simulink model "ET223104_complex_lab"  (R2023a)
settings: Solver=VariableStepAuto  StartTime=0.0  StopTime=10.0  RelTol=1e-3
libraries: spsThreePhaseSeriesRLCBranchLib x10, spsLoadFlowBusLib x9, spsThreePhaseVIMeasurementLib x9, spsThreePhaseParallelRLCLoadLib x6, spsThreePhaseSourceLib x3, sps_lib x1
settings Model: Creator=shahrearhossain  LastModifiedBy=shahrearhossain

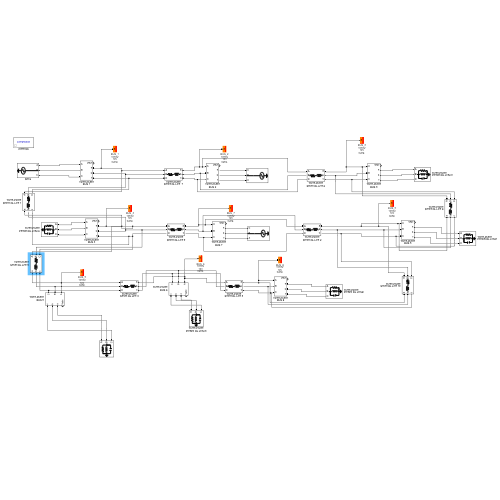
[thumbnail: Simulink's stored preview of the top-level diagram]
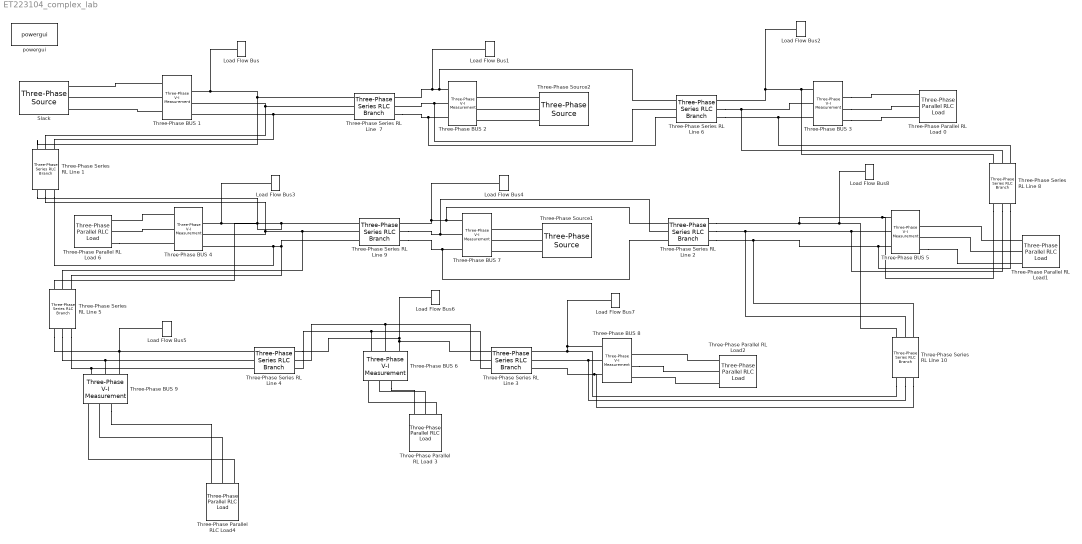
== system ET223104_complex_lab ==
  Load Flow Bus : spsLoadFlowBusLib/Load Flow Bus  LConnTagsString=a  Phases=single  Connectors=on one side  ID=BUS_1  Vbase=10e3  Vref=1.0  Vangle=0  VLF=1  VLFb=1  VLFc=1  angleLF=0  angleLFb=0  angleLFc=0
  Load Flow Bus1 : spsLoadFlowBusLib/Load Flow Bus  LConnTagsString=a  Phases=single  Connectors=on one side  ID=BUS_2  Vbase=10e3  Vref=1.05  Vangle=0  VLF=1  VLFb=1  VLFc=1  angleLF=0  angleLFb=0  angleLFc=0
  Load Flow Bus2 : spsLoadFlowBusLib/Load Flow Bus  LConnTagsString=a  Phases=single  Connectors=on one side  ID=BUS_3  Vbase=10e3  Vref=1.05  Vangle=0  VLF=1  VLFb=1  VLFc=1  angleLF=0  angleLFb=0  angleLFc=0
  Load Flow Bus3 : spsLoadFlowBusLib/Load Flow Bus  LConnTagsString=a  Phases=single  Connectors=on one side  ID=BUS_4  Vbase=10e3  Vref=1.05  Vangle=0  VLF=1  VLFb=1  VLFc=1  angleLF=0  angleLFb=0  angleLFc=0
  Load Flow Bus4 : spsLoadFlowBusLib/Load Flow Bus  LConnTagsString=a  Phases=single  Connectors=on one side  ID=BUS_7  Vbase=10e3  Vref=1.05  Vangle=0  VLF=1  VLFb=1  VLFc=1  angleLF=0  angleLFb=0  angleLFc=0
  Load Flow Bus5 : spsLoadFlowBusLib/Load Flow Bus  LConnTagsString=a  Phases=single  Connectors=on one side  ID=BUS_9  Vbase=10e3  Vref=1.05  Vangle=0  VLF=1  VLFb=1  VLFc=1  angleLF=0  angleLFb=0  angleLFc=0
  Load Flow Bus6 : spsLoadFlowBusLib/Load Flow Bus  LConnTagsString=a  Phases=single  Connectors=on one side  ID=BUS_6  Vbase=10e3  Vref=1.05  Vangle=0  VLF=1  VLFb=1  VLFc=1  angleLF=0  angleLFb=0  angleLFc=0
  Load Flow Bus7 : spsLoadFlowBusLib/Load Flow Bus  LConnTagsString=a  Phases=single  Connectors=on one side  ID=BUS_8  Vbase=10e3  Vref=1.05  Vangle=0  VLF=1  VLFb=1  VLFc=1  angleLF=0  angleLFb=0  angleLFc=0
  Load Flow Bus8 : spsLoadFlowBusLib/Load Flow Bus  LConnTagsString=a  Phases=single  Connectors=on one side  ID=BUS_5  Vbase=10e3  Vref=1.05  Vangle=0  VLF=1  VLFb=1  VLFc=1  angleLF=0  angleLFb=0  angleLFc=0
  Slack : spsThreePhaseSourceLib/Three-Phase Source  InternalConnection=Yg  VoltagePhases=off  Voltage=10e3  PhaseAngle=0  Voltage_phases=[25e3 25e3 25e3]/sqrt(3)  PhaseAngles_phases=[0 -120 +120]  Frequency=60  NonIdealSource=off  SpecifyImpedance=off  Resistance=0.8929  Inductance=16.58e-3  ShortCircuitLevel=100e6  BaseVoltage=25e3  XRratio=7  BusType=swing  Pref=40e6  Qref=20e6  Prefabc=[10e3, 10e3, 10e3]  Qrefabc=[0, 0, 0]  Qmin=-inf  Qmax=inf
  Three-Phase BUS {1..9} (9 alike) : spsThreePhaseVIMeasurementLib/Three-Phase V-I Measurement  VoltageMeasurement=phase-to-phase  SetLabelV=off  LabelV=Vabc  Vpu=off  VpuLL=off  CurrentMeasurement=no  SetLabelI=off  LabelI=Iabc  Ipu=off  Pbase=100e6  Vbase=500e3  OutputType=Complex  PhasorSimulation=off  PSBequivalent=0
  Three-Phase Parallel RL Load 0 : spsThreePhaseParallelRLCLoadLib/Three-Phase Parallel RLC Load  LConnTagsString=A|B|C  Configuration=Y (grounded)  NominalVoltage=10000  Vabc=[1e3 1e3 1e3]  Vabcp=[1e3 1e3 1e3]  NominalFrequency=60  UnbalancedPower=off  ActivePower=110e6  InductivePower=12e6  CapacitivePower=100  Pabc=[10e3 9e3 11e3]  QLabc=[100 90 110]  QCabc=[100 90 110]  Pabcp=[10e3 9e3 11e3]  QLabcp=[100 90 110]  QCabcp=[100 90 110]  Measurements=None  LoadType=constant PQ
  Three-Phase Parallel RL Load 3 : spsThreePhaseParallelRLCLoadLib/Three-Phase Parallel RLC Load  LConnTagsString=A|B|C  Configuration=Y (grounded)  NominalVoltage=10000  Vabc=[1e3 1e3 1e3]  Vabcp=[1e3 1e3 1e3]  NominalFrequency=60  UnbalancedPower=off  ActivePower=110e6  InductivePower=12e6  CapacitivePower=100  Pabc=[10e3 9e3 11e3]  QLabc=[100 90 110]  QCabc=[100 90 110]  Pabcp=[10e3 9e3 11e3]  QLabcp=[100 90 110]  QCabcp=[100 90 110]  Measurements=None  LoadType=constant PQ
  Three-Phase Parallel RL Load 6 : spsThreePhaseParallelRLCLoadLib/Three-Phase Parallel RLC Load  LConnTagsString=A|B|C  Configuration=Y (grounded)  NominalVoltage=10000  Vabc=[1e3 1e3 1e3]  Vabcp=[1e3 1e3 1e3]  NominalFrequency=60  UnbalancedPower=off  ActivePower=110e6  InductivePower=12e6  CapacitivePower=100  Pabc=[10e3 9e3 11e3]  QLabc=[100 90 110]  QCabc=[100 90 110]  Pabcp=[10e3 9e3 11e3]  QLabcp=[100 90 110]  QCabcp=[100 90 110]  Measurements=None  LoadType=constant PQ
  Three-Phase Parallel RL Load1 : spsThreePhaseParallelRLCLoadLib/Three-Phase Parallel RLC Load  LConnTagsString=A|B|C  Configuration=Y (grounded)  NominalVoltage=10000  Vabc=[1e3 1e3 1e3]  Vabcp=[1e3 1e3 1e3]  NominalFrequency=60  UnbalancedPower=off  ActivePower=110e6  InductivePower=12e6  CapacitivePower=100  Pabc=[10e3 9e3 11e3]  QLabc=[100 90 110]  QCabc=[100 90 110]  Pabcp=[10e3 9e3 11e3]  QLabcp=[100 90 110]  QCabcp=[100 90 110]  Measurements=None  LoadType=constant PQ
  Three-Phase Parallel RL Load2 : spsThreePhaseParallelRLCLoadLib/Three-Phase Parallel RLC Load  LConnTagsString=A|B|C  Configuration=Y (grounded)  NominalVoltage=10000  Vabc=[1e3 1e3 1e3]  Vabcp=[1e3 1e3 1e3]  NominalFrequency=60  UnbalancedPower=off  ActivePower=110e6  InductivePower=12e6  CapacitivePower=100  Pabc=[10e3 9e3 11e3]  QLabc=[100 90 110]  QCabc=[100 90 110]  Pabcp=[10e3 9e3 11e3]  QLabcp=[100 90 110]  QCabcp=[100 90 110]  Measurements=None  LoadType=constant PQ
  Three-Phase Parallel RLC Load4 : spsThreePhaseParallelRLCLoadLib/Three-Phase Parallel RLC Load  LConnTagsString=A|B|C  Configuration=Y (grounded)  NominalVoltage=10000  Vabc=[1e3 1e3 1e3]  Vabcp=[1e3 1e3 1e3]  NominalFrequency=60  UnbalancedPower=off  ActivePower=110e6  InductivePower=12e6  CapacitivePower=100  Pabc=[10e3 9e3 11e3]  QLabc=[100 90 110]  QCabc=[100 90 110]  Pabcp=[10e3 9e3 11e3]  QLabcp=[100 90 110]  QCabcp=[100 90 110]  Measurements=None  LoadType=constant PQ
  Three-Phase Series RL LIne 10 : spsThreePhaseSeriesRLCBranchLib/Three-Phase Series RLC Branch  LConnTagsString=A|B|C  RConnTagsString=A|B|C  BranchType=RL  Resistance=0.02*1  Inductance=0.04*1/(2*3.14*60)  Capacitance=1e-6  Measurements=None
  Three-Phase Series RL Line  7 : spsThreePhaseSeriesRLCBranchLib/Three-Phase Series RLC Branch  LConnTagsString=A|B|C  RConnTagsString=A|B|C  BranchType=RL  Resistance=0.02*1  Inductance=0.04*1/(2*3.14*60)  Capacitance=1e-6  Measurements=None
  Three-Phase Series RL Line {1..6,8..9} (8 alike) : spsThreePhaseSeriesRLCBranchLib/Three-Phase Series RLC Branch  LConnTagsString=A|B|C  RConnTagsString=A|B|C  BranchType=RL  Resistance=0.02*1  Inductance=0.04*1/(2*3.14*60)  Capacitance=1e-6  Measurements=None
  Three-Phase Source1 : spsThreePhaseSourceLib/Three-Phase Source  InternalConnection=Yg  VoltagePhases=off  Voltage=10e3  PhaseAngle=0  Voltage_phases=[25e3 25e3 25e3]/sqrt(3)  PhaseAngles_phases=[0 -120 +120]  Frequency=60  NonIdealSource=off  SpecifyImpedance=off  Resistance=0.8929  Inductance=16.58e-3  ShortCircuitLevel=100e6  BaseVoltage=25e3  XRratio=7  BusType=PQ  Pref=40e6  Qref=20e6  Prefabc=[10e3, 10e3, 10e3]  Qrefabc=[0, 0, 0]  Qmin=-inf  Qmax=inf
  Three-Phase Source2 : spsThreePhaseSourceLib/Three-Phase Source  InternalConnection=Yg  VoltagePhases=off  Voltage=10e3  PhaseAngle=0  Voltage_phases=[25e3 25e3 25e3]/sqrt(3)  PhaseAngles_phases=[0 -120 +120]  Frequency=60  NonIdealSource=off  SpecifyImpedance=off  Resistance=0.8929  Inductance=16.58e-3  ShortCircuitLevel=100e6  BaseVoltage=25e3  XRratio=7  BusType=PQ  Pref=40e6  Qref=20e6  Prefabc=[10e3, 10e3, 10e3]  Qrefabc=[0, 0, 0]  Qmin=-inf  Qmax=inf
  powergui : sps_lib/powergui  Priority=1  SimulationMode=Continuous  SampleTime=50e-6  frequency=60  Iterations=50  frequencyindice=60  Pbase=100e6  ErrMax=1e-4  UnitsV=kV  UnitsW=MW  buscounter=0  FunctionMessages=off  echomessages=off  EnableUseOfTLC=off  CurrentSourceSwitches=off  DisableSnubberDevices=off  DisableRonSwitches=off  DisableVfSwitches=off  DisplayEquations=off  AutomaticDiscreteSolvers=off  SolverType=Tustin/Backward Euler (TBE)  Interpol=off  ExternalGateDelay=off  methode=off  Ts=100  x0status=blocks  SPID=on  SwTol=0  HookPort=off  NonlinearTolerance=1e-4  nMaxIteration=100  ContinueOnMaxIteration=off  RestoreLinks=warning  ResistiveCurrentMeasurement=off  Frange=[0:2:500]  Ylog=off  Xlog=on  ShowGrid=off  save=off  variable=ZData  structure=0  ZoomFFT=off  StartTime=0.0  cycles=1  DisplayStyle=1  fundamental=60  FreqAxis=off  MaxFrequency=1000  frequencyindicesteady=1  RmsSteady=1  display=off
  connections:
  Three-Phase BUS 1/LConn1 -- Slack/RConn1
  Three-Phase BUS 1/LConn3 -- Slack/RConn3
  Three-Phase BUS 1/LConn2 -- Slack/RConn2
  Three-Phase BUS 4/LConn1 -- Three-Phase Parallel RL Load 6/LConn1
  Three-Phase BUS 4/LConn2 -- Three-Phase Parallel RL Load 6/LConn2
  Three-Phase Parallel RL Load 6/LConn3 -- Three-Phase BUS 4/LConn3
  Three-Phase BUS 2/LConn1 -- Three-Phase Series RL Line 6/LConn1 -- Load Flow Bus1/LConn1 -- Three-Phase Series RL Line  7/RConn1
  Three-Phase BUS 2/LConn2 -- Three-Phase Series RL Line 6/LConn2 -- Three-Phase Series RL Line  7/RConn2
  Three-Phase Series RL Line  7/RConn3 -- Three-Phase Series RL Line 6/LConn3 -- Three-Phase BUS 2/LConn3
  Three-Phase BUS 3/LConn1 -- Load Flow Bus2/LConn1 -- Three-Phase Series RL Line 6/RConn1 -- Three-Phase Series RL Line 8/LConn1
  Three-Phase Series RL Line 6/RConn2 -- Three-Phase Series RL Line 8/LConn2 -- Three-Phase BUS 3/LConn2
  Three-Phase Series RL Line 6/RConn3 -- Three-Phase Series RL Line 8/LConn3 -- Three-Phase BUS 3/LConn3
  Three-Phase BUS 3/RConn1 -- Three-Phase Parallel RL Load 0/LConn1
  Three-Phase BUS 3/RConn2 -- Three-Phase Parallel RL Load 0/LConn2
  Three-Phase BUS 3/RConn3 -- Three-Phase Parallel RL Load 0/LConn3
  Three-Phase Parallel RL Load1/LConn1 -- Three-Phase BUS 5/RConn1
  Three-Phase Parallel RL Load1/LConn2 -- Three-Phase BUS 5/RConn2
  Three-Phase BUS 5/RConn3 -- Three-Phase Parallel RL Load1/LConn3
  Three-Phase BUS 9/RConn1 -- Three-Phase Parallel RLC Load4/LConn1
  Three-Phase Parallel RLC Load4/LConn2 -- Three-Phase BUS 9/RConn2
  Three-Phase Parallel RLC Load4/LConn3 -- Three-Phase BUS 9/RConn3
  Three-Phase BUS 6/RConn1 -- Three-Phase Parallel RL Load 3/LConn1
  Three-Phase Parallel RL Load 3/LConn2 -- Three-Phase BUS 6/RConn2
  Three-Phase Parallel RL Load 3/LConn3 -- Three-Phase BUS 6/RConn3
  Three-Phase Parallel RL Load2/LConn1 -- Three-Phase BUS 8/RConn1
  Three-Phase BUS 8/RConn2 -- Three-Phase Parallel RL Load2/LConn2
  Three-Phase Parallel RL Load2/LConn3 -- Three-Phase BUS 8/RConn3
  Three-Phase Series RL Line  7/LConn1 -- Three-Phase Series RL Line 1/LConn1 -- Load Flow Bus/LConn1 -- Three-Phase BUS 1/RConn1
  Three-Phase Series RL Line  7/LConn2 -- Three-Phase Series RL Line 1/LConn2 -- Three-Phase BUS 1/RConn2
  Three-Phase Series RL Line  7/LConn3 -- Three-Phase Series RL Line 1/LConn3 -- Three-Phase BUS 1/RConn3
  Three-Phase Series RL Line 9/LConn1 -- Three-Phase Series RL Line 5/LConn1 -- Three-Phase Series RL Line 1/RConn1 -- Load Flow Bus3/LConn1 -- Three-Phase BUS 4/RConn1
  Three-Phase Series RL Line 9/LConn2 -- Three-Phase Series RL Line 5/LConn2 -- Three-Phase Series RL Line 1/RConn2 -- Three-Phase BUS 4/RConn2
  Three-Phase Series RL Line 9/LConn3 -- Three-Phase Series RL Line 5/LConn3 -- Three-Phase Series RL Line 1/RConn3 -- Three-Phase BUS 4/RConn3
  Three-Phase BUS 7/LConn1 -- Three-Phase Series RL Line 2/LConn1 -- Load Flow Bus4/LConn1 -- Three-Phase Series RL Line 9/RConn1
  Three-Phase Series RL Line 9/RConn2 -- Three-Phase Series RL Line 2/LConn2 -- Three-Phase BUS 7/LConn2
  Three-Phase Series RL Line 9/RConn3 -- Three-Phase Series RL Line 2/LConn3 -- Three-Phase BUS 7/LConn3
  Three-Phase Series RL Line 2/RConn1 -- Load Flow Bus8/LConn1 -- Three-Phase Series RL LIne 10/LConn1 -- Three-Phase Series RL Line 8/RConn1 -- Three-Phase BUS 5/LConn1
  Three-Phase Series RL Line 2/RConn2 -- Three-Phase Series RL LIne 10/LConn2 -- Three-Phase Series RL Line 8/RConn2 -- Three-Phase BUS 5/LConn2
  Three-Phase Series RL Line 2/RConn3 -- Three-Phase Series RL Line 8/RConn3 -- Three-Phase BUS 5/LConn3 -- Three-Phase Series RL LIne 10/LConn3
  Three-Phase Series RL Line 4/RConn1 -- Three-Phase BUS 6/LConn1 -- Three-Phase Series RL Line 3/LConn1 -- Load Flow Bus6/LConn1
  Three-Phase BUS 6/LConn2 -- Three-Phase Series RL Line 4/RConn2 -- Three-Phase Series RL Line 3/LConn2
  Three-Phase BUS 6/LConn3 -- Three-Phase Series RL Line 3/LConn3 -- Three-Phase Series RL Line 4/RConn3
  Three-Phase BUS 8/LConn1 -- Load Flow Bus7/LConn1 -- Three-Phase Series RL Line 3/RConn1 -- Three-Phase Series RL LIne 10/RConn1
  Three-Phase BUS 8/LConn2 -- Three-Phase Series RL Line 3/RConn2 -- Three-Phase Series RL LIne 10/RConn2
  Three-Phase BUS 8/LConn3 -- Three-Phase Series RL Line 3/RConn3 -- Three-Phase Series RL LIne 10/RConn3
  Three-Phase Series RL Line 4/LConn1 -- Three-Phase Series RL Line 5/RConn1 -- Three-Phase BUS 9/LConn1 -- Load Flow Bus5/LConn1
  Three-Phase Series RL Line 4/LConn2 -- Three-Phase Series RL Line 5/RConn2 -- Three-Phase BUS 9/LConn2
  Three-Phase Series RL Line 4/LConn3 -- Three-Phase Series RL Line 5/RConn3 -- Three-Phase BUS 9/LConn3
  Three-Phase Source1/RConn3 -- Three-Phase BUS 7/RConn1
  Three-Phase Source1/RConn2 -- Three-Phase BUS 7/RConn2
  Three-Phase Source1/RConn1 -- Three-Phase BUS 7/RConn3
  Three-Phase Source2/RConn3 -- Three-Phase BUS 2/RConn1
  Three-Phase Source2/RConn2 -- Three-Phase BUS 2/RConn2
  Three-Phase Source2/RConn1 -- Three-Phase BUS 2/RConn3
